simulink model "TransmissionController"  (R2026a)
settings: Solver=FixedStepAuto  StopTime=65  FixedStep=0.01
undefined symbols (not defined in the file): RangeSelected
libraries: simulink x7, sl_discontinuities x1
settings Model: DataDictionary=ETRS_data.sldd  Creator=macec  LastModifiedBy=Prest

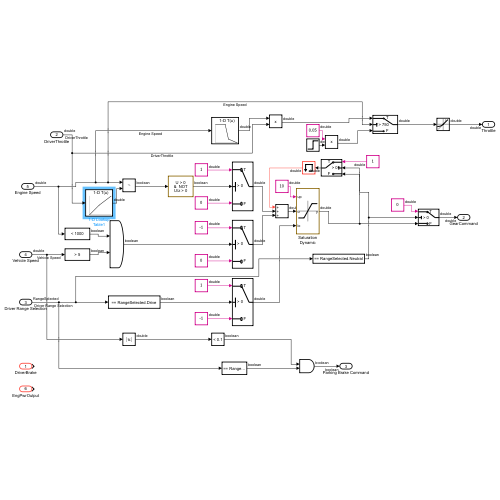
[thumbnail: Simulink's stored preview of the top-level diagram]
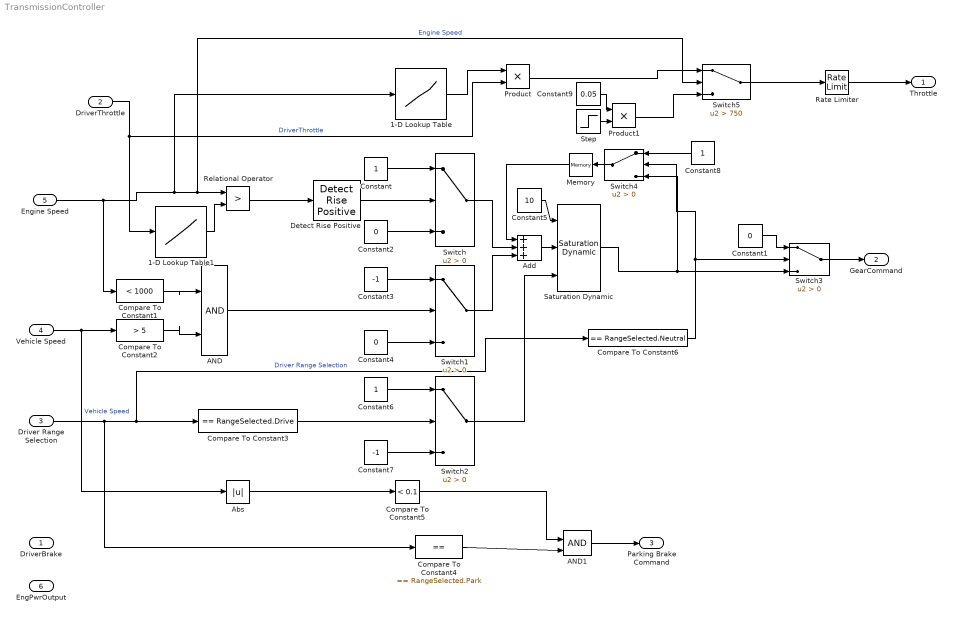
== system TransmissionController ==
  DriverBrake : Inport  OutDataTypeStr=double  PortDimensions=1
  DriverThrottle : Inport  Port=2  OutDataTypeStr=double  PortDimensions=1
  Driver Range Selection : Inport  Port=3  OutDataTypeStr=Enum: RangeSelected  PortDimensions=1
  Vehicle Speed : Inport  Port=4  OutDataTypeStr=double  PortDimensions=1
  Engine Speed : Inport  Port=5  OutDataTypeStr=double  PortDimensions=1
  EngPwrOutput : Inport  Port=6
  1-D Lookup Table : Lookup_n-D  NumberOfTableDimensions=1  BreakpointsForDimension1=[0, 4500, 6000, 10000]  Table=[1, 1, 0.2, 0]  ExtrapMethod=Clip  InternalRulePriority=Speed  RndMeth=Simplest
  1-D Lookup Table1 : Lookup_n-D  NumberOfTableDimensions=1  BreakpointsForDimension1=[0.1, 0.5, 1.0]  Table=[2000, 4000, 6000]  InternalRulePriority=Speed  RndMeth=Simplest
  AND : Logic  IconShape=distinctive  AllPortsSameDT=off  OutDataTypeStr=boolean
  AND1 : Logic  IconShape=distinctive  AllPortsSameDT=off  OutDataTypeStr=boolean
  Abs : Abs  SaturateOnIntegerOverflow=off
  Add : Sum  Inputs=+++
  Compare To Constant1 : simulink/Logic and Bit Operations/Compare To Constant  relop=<  const=1000  OutDataTypeStr=boolean
  Compare To Constant2 : simulink/Logic and Bit Operations/Compare To Constant  relop=>  const=5  OutDataTypeStr=boolean
  Compare To Constant3 : simulink/Logic and Bit Operations/Compare To Constant  relop===  const=RangeSelected.Drive  OutDataTypeStr=boolean
  Compare To Constant4 : simulink/Logic and Bit Operations/Compare To Constant  relop===  const=RangeSelected.Park  OutDataTypeStr=boolean
  Compare To Constant5 : simulink/Logic and Bit Operations/Compare To Constant  relop=<  const=0.1  OutDataTypeStr=boolean
  Compare To Constant6 : simulink/Logic and Bit Operations/Compare To Constant  relop===  const=RangeSelected.Neutral  OutDataTypeStr=boolean
  Constant : Constant
  Constant1 : Constant  Value=0
  Constant2 : Constant  Value=0
  Constant3 : Constant  Value=-1
  Constant4 : Constant  Value=0
  Constant5 : Constant  Value=10
  Constant6 : Constant
  Constant7 : Constant  Value=-1
  Constant8 : Constant
  Constant9 : Constant  Value=0.05
  Detect Rise Positive : simulink/Logic and Bit Operations/Detect Rise Positive  vinit=0  OutDataTypeStr=boolean
  Memory : Memory  InheritSampleTime=on
  Product : Product
  Product1 : Product
  Rate Limiter : RateLimiter  RisingSlewLimit=2  FallingSlewLimit=-5  SampleTimeMode=inherited
  Relational Operator : RelationalOperator  Operator=>  OutDataTypeStr=boolean  RndMeth=Simplest  InputSameDT=off
  Saturation Dynamic : sl_discontinuities/Saturation Dynamic  OutMin=[]  OutMax=[]  OutDataTypeStr=Inherit: Same as second input  OutDataType=fixdt(1, 16)  OutScaling=2^-10  DoSatur=off
      settings: LibrarySourceBlock=|
      | simulink/Discontinuities/Saturation
      | Dynamic
  Step : Step  Time=0.1  SampleTime=0
  Switch{,1..4} (5 alike) : Switch  Criteria=u2 > Threshold  SaturateOnIntegerOverflow=off  InputSameDT=off
  Switch5 : Switch  Criteria=u2 > Threshold  Threshold=750  SaturateOnIntegerOverflow=off  InputSameDT=off
  Throttle : Outport  OutDataTypeStr=double  PortDimensions=1
  GearCommand : Outport  Port=2  OutDataTypeStr=double  PortDimensions=1
  Parking Brake Command : Outport  Port=3  OutDataTypeStr=boolean  PortDimensions=1
  wires:
  Driver Range Selection/1 -> Compare To Constant4/1, Compare To Constant6/1, Compare To Constant3/1  "Driver Range Selection"
  Vehicle Speed/1 -> Abs/1, Compare To Constant2/1  "Vehicle Speed"
  Engine Speed/1 -> 1-D Lookup Table/1, Switch5/2, Relational Operator/1, Compare To Constant1/1  "Engine Speed"
  Constant/1 -> Switch/1
  Constant2/1 -> Switch/3
  Constant3/1 -> Switch1/1
  Constant4/1 -> Switch1/3
  Compare To Constant2/1 -> AND/2
  AND/1 -> Switch1/2
  Compare To Constant1/1 -> AND/1
  Switch1/1 -> Add/3
  Switch/1 -> Add/2
  Memory/1 -> Add/1
  Constant5/1 -> Saturation Dynamic/1
  Add/1 -> Saturation Dynamic/2
  Constant6/1 -> Switch2/1
  Constant7/1 -> Switch2/3
  Switch2/1 -> Saturation Dynamic/3
  DriverThrottle/1 -> 1-D Lookup Table1/1, Product/2  "DriverThrottle"
  Abs/1 -> Compare To Constant5/1
  Compare To Constant4/1 -> AND1/2
  Compare To Constant5/1 -> AND1/1
  AND1/1 -> Parking Brake Command/1
  Compare To Constant3/1 -> Switch2/2
  Compare To Constant6/1 -> Switch4/2, Switch3/2
  Constant1/1 -> Switch3/1
  Switch3/1 -> GearCommand/1
  1-D Lookup Table/1 -> Product/1
  Detect Rise Positive/1 -> Switch/2
  Relational Operator/1 -> Detect Rise Positive/1
  Switch4/1 -> Memory/1
  Constant8/1 -> Switch4/1
  1-D Lookup Table1/1 -> Relational Operator/2
  Product/1 -> Switch5/1
  Switch5/1 -> Rate Limiter/1
  Step/1 -> Product1/2
  Product1/1 -> Switch5/3
  Constant9/1 -> Product1/1
  Rate Limiter/1 -> Throttle/1
  Saturation Dynamic/1 -> Switch4/3, Switch3/3
